simulink model "Example_SOMU_SYNC"  (R2018b)
settings: Solver=FixedStepDiscrete  StartTime=0.0  StopTime=inf  RelTol=1e-3  EnableMultiTasking=on
model workspace: external: MATLAB File (data not in the file)
values from neighbouring files (symbols this model uses):
  kT = acker(Ad,bd,[0.8,0.6])    [aaass.m]
  numOfObj = 5    [aaass.m]    (also in followerGUI.m = max(1,block.DialogPrm(1).Data))
  Td = 0.5    [aaass.m]    (also in controllerSpeed.m = block.DialogPrm(2).Data; followerGUI.m = block.DialogPrm(2).Data; leaderGUI.m = block.DialogPrm(2).Data)
  V = 1./(cT*inv(eye*(2) - Ad+bd*kT)*bd)    [aaass.m]
undefined symbols (not defined in the file or in its folder): Lib_SUMOInterface, MPCController1, sigbuilder_block, SUMU_SIMULINK_SYNC
libraries: simulink x2, Lib_SENSOR x1
settings Model: Creator=michaelstolz  LastModifiedBy=HP
settings SolverCC: AlgebraicLoopSolver=LineSearch
settings DataIOCC: SaveFormat=Array  SaveOutput=off  SignalLogging=off  SaveTime=off
settings OptimizationCC: LifeSpan=inf
settings DebuggingCC: UnderspecifiedInitializationDetection=Classic  MergeDetectMultiDrivingBlocksExec=none  SolverPrmCheckMsg=warning  FcnCallInpInsideContextMsg=warning  SFUnexpectedBacktrackingDiag=warning  SFNoUnconditionalDefaultTransitionDiag=warning  SFExecutionAtInitializationDiag=none
settings HardwareCC: ProdBitPerPointer=32  ProdBitPerSizeT=32  ProdBitPerPtrDiffT=32  ProdLargestAtomicFloat=None  ProdIntDivRoundTo=Undefined  ProdEndianess=Unspecified  ProdWordSize=32  ProdHWDeviceType=32-bit Generic
settings ModelReferenceCC: PropagateSignalLabelsOutOfModel=off
settings SFSimCC: SimUseLocalCustomCode=off
settings RTWCC: RTWUseLocalCustomCode=off
settings CodeAppCC: StateflowObjectComments=on
settings GRTTargetCC: TargetLangStandard=C89/C90 (ANSI)  GeneratePreprocessorConditionals=Disable all
settings ConfigComp: CovMetricSettings=dw  CovHtmlReporting=on  CovSaveCumulativeToWorkspaceVar=on  CovSaveSingleToWorkspaceVar=on  CovExternalEMLEnable=off

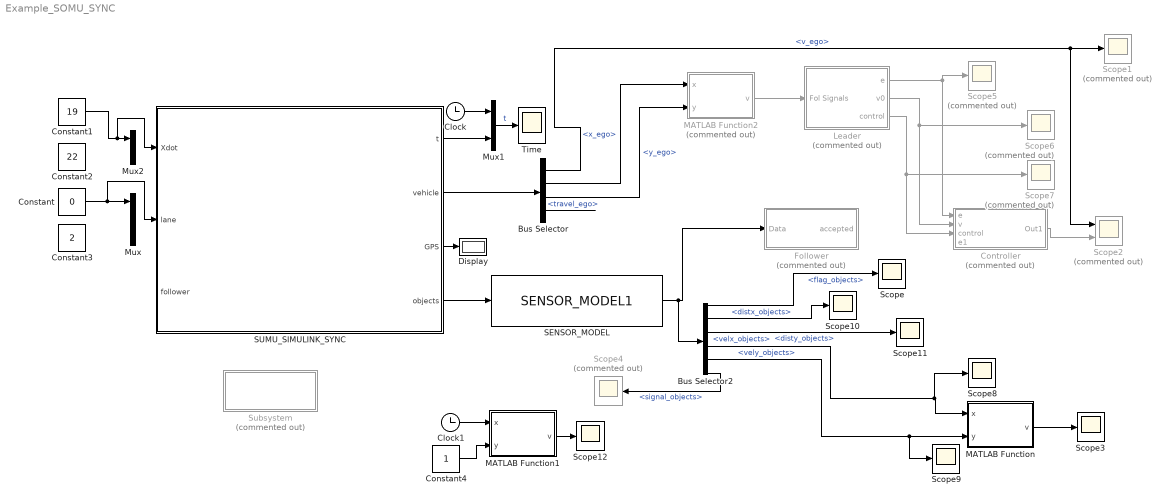
== system Example_SOMU_SYNC ==
  Bus Selector : BusSelector  OutputSignals=v_ego,x_ego,y_ego,travel_ego
  Bus Selector2 : BusSelector  OutputSignals=flag_objects,distx_objects,disty_objects,velx_objects,vely_objects,signal_objects
  Clock : Clock
  Clock1 : Clock
  Constant : Constant  Value=0
  Constant1 : Constant  Value=19
  Constant2 : Constant  Value=22
  Constant3 : Constant  Value=2
  Constant4 : Constant
  Controller : Subsystem  Commented=on
  Display : Display
  Follower : Subsystem  Commented=on
  Leader : Subsystem  Commented=on
  MATLAB Function : MATLAB Function  TreatAsAtomicUnit=on
  MATLAB Function1 : MATLAB Function  TreatAsAtomicUnit=on
  MATLAB Function2 : MATLAB Function  Commented=on  TreatAsAtomicUnit=on
  Mux : Mux  Inputs=3
  Mux1 : Mux  Inputs=2
  Mux2 : Mux  Inputs=3
  SENSOR_MODEL : Lib_SENSOR/SENSOR_MODEL1  NumObjects_=numOfObj  MountX_=[-4,-2,-2]  MountY_=[0,1,-1]  MountA_=[180,90,-90]  SensorModel_=Sector Model  SensorAngle_=[80,100,100]  SensorRange_=[200,20,20]  SensorXY_="{[0   6.5  12.5  20 27.5  35  42.5 47.5 41;  0   7  12  16 19 20  19 10 0 ], [0   6.5  12.5  20 27.5  35  42.5 47.5 41;  0   7  12  16 19 20  19 10 0 ], [0   6.5  12.5  20 27.5  35  42.5 47.5 41;  0   7  12  16 19 20  19 10 0 ]}"  SensorVisibility_=Segmentation  SensorSegmentation_=50  SensorMinVis_=0  SensorType_={'L','L','R'}  NrSensors_=1
  SUMU_SIMULINK_SYNC : Subsystem  AncestorBlock=Lib_SUMOInterface/SUMU_SIMULINK_SYNC  mask(SUMO Simulink Syncronisation){SumoTs_=Td, EgoName_={'ego'}, SumoCfg_=data1\hokkaido.sumocfg, SumoGui_=on, SumoIP_=127.0.0.1, SumoPort_=8873, SumoOptions_=, NumVehicles_=numOfObj, SensorRange_=500, NumTLights_=2}
      mask prompts: SumoTs_ "Sample time for SUMO in [s]"; EgoName_ "Ego vehicle name(s) in SUMO"; SumoCfg_ "SUMO config-file name. (delete for dialog)"; SumoGui_ "Select if the GUI is used or the command line executable."; SumoIP_ "Connection name (default '127.0.0.1')"; SumoPort_ "Port number for SUMO connection (deault 8873)."; SumoOptions_ "Additional command line options for sumo executable."; NumVehicles_ "Maximum number of traffic objects"; SensorRange_ "Detection range [m]. (values <=0 disables range checking)"; NumTLights_ "Maximum number of traffic lights"
      mask help:
      | This Block syncs a vehicle simulation in Simulink with a traffic simulation
      | in SUMO.
      |
      | Syncronisation is performed for one or more vehicle(s) called the
      | "ego"-vehicle(s).
      | The position and velocity information provided from vehicle simulation is
      | send to SUMO to move the corresponding vehicle in the traffic simulation
      | acordingly.
      |
      | Inputs:
      | X     [m] ...... horzintal position of vehicle to sync
      | Y     [m] ...... vertical position of vehicle to sync
      | dX/dt [m/s] .... horizontal velocity of vehicle to sync
      | dY/dt [m/s] .... horizontal velocity of vehicle to sync
      | T     [rad] .... orientation of vehicle to sync
      |                  ( OPTIONAL if sensors are used, otherwise set to NaN )
      | lane  [-] ...... lane of vehicle if in a multilane scenario
      |                  ( currently not used )
      | y_L   [m] ...... lateral offset of vehicle to sync
      |                  ( OPTIONAL if lane assignment shall be done, otherwise 0)
      |
      | Outputs:
      |  * t [s] ....... SUMO simulation time
      |                  (for checking and for traffic light trigger checks)
      |  * vehicle ..... information for ego vehicle(s) within a bus
      |  * GPS   ....... additional GPS information for ego vehicle(s) in a bus
      |  * objects ..... information regarding traffic objects in range in a bus
      |  * signals ..... information regarding traffic lights ahead in a bus
      |
      | Please read the help text for further information.
      mask Help:
      | MASK PARAMETERS:
      | 
      | The following mask parameters can be set, in order to control the behavior of the sync interface:
      | 
      | o) Ego vehicle names as strings in cell array. These names correspond to to the vehicle names in the SUMO config file which should be synced.
      | o) SUMO sample time in [s]: this is the fixed time step SUMO is updated
      | o) SUMO interface IP adress and port number
      | o) SUMO graphical mode activation/diactivation: set wheter to use the gui or command line tool only
      | o) SUMO configuartion file name: better use relative paths for interoperability
      | o) SUMO additional command line parameters: add options to e.g. log something
      | 
      | o) Maximum number of traffic objects to be send at output
      | o) Maximum range around vehicle for traffic objects to be relevant
      | 
      | o) Maximum number of traffic lights to be send at output
      | 
      | POSITION SYNCRONISATION:
      | 
      | Due to several shortcomings of the used TraCi-Interface from SUMO direct position synchronization could not be used in general, therefore
      | indirect synchronization via velocity is used.
      | 
      | Velocity information is used as main syncronization method. Position info is used additionally to correct velocity to improve matching and avoid
      | drifting.
      | Note that setting velocity of the ego-vehicle for synchronization will not in all cases take imidiate effect due to acceleration limits and driver
      | model limitations. However a lot of measures have been taken in order to set the velocity directly:
      |   * min/max acceleration rates have been set to +-1000
      |   * time const of driver model has been set to 0
      |   * speed mode has been set to 0 --> ignoring a lot of speedlimits
      |   * --ignore-accidents has been used in command line
      | 
      | 
      | 
      | INTERFACES:
      | 
      | t : scalar time of SUMO-simulation in seconds.
      | 
      | vehicle : a bus holding ego vehicles informations
      |     * X position [m]
      |     * Y position [m]
      |     * V velocity [m/s]
      |     * T angle [rad] (anticlockwise starting from x)
      |     * D traveled distance [m]
      | 
      | GPS: a bus holding information from FIRST ego car and its road segment
      | 
      | objects: a bus holding information from traffic objects in the given range (mask parameter) of the FIRST ego car. Note the bus signals stay the same, the dimension of each signal will depend on the selected maximum number of traffic objects (mask parameter)
      |  flag_objects : 0=off, 1=on, 2=on and new
      | distx_objects : the distance of the object measured in coordinate system of the FIRST ego vehicle along the x axis
      | disty_objects : the distance of the object measured in coordinate system of the FIRST ego vehicle along the y axis
      | velx_objects : the velocity (absolute!) of the object measured in coordinate system of the FIRST ego vehicle along the x axis
      | vely_objects : the velocity (absolute!) of the object measured in coordinate system of the FIRST ego vehicle along the y axis
      | signal_objects : the signal state of the traffic object. see SUMO documentation for details (brake signal, lane change signal, ...)
      | 
      | signals: a bus holding information from traffic lights ahead of the FIRST ego vehicle. Note the bus signals stay the same, the dimension of each signal will depend on the selected maximum number of traffic lights (mask parameter).
      | flag_signals     : 0=off, 1=on
      | distance_signals : driving distance along the road to the traffic light
      | tswitch_signals  : (absolute) time instance of next switching in seconds
      | phase_signals    : current phase (0 for green, 1 for red)
      | red_signals      : duration of red phase in seconds
      | green_signals    : duration of green phase in seconds
      mask TypeOptions SumoTs_: SIM_SYNC/SumoTs
      mask TypeOptions EgoName_: SIM_SYNC/EgoName
      mask Callback EgoName_:
      | if isempty(get_param(gcb,'EgoName_')),
      |     set_param(gcb, 'EgoName_','{''ego''}');
      | end
      mask TypeOptions SumoCfg_: SIM_SYNC/SumoCfg
      mask Callback SumoCfg_:
      | if isempty(get_param(gcb,'SumoCfg_')),
      |     [myvars.fileName, myvars.filePath] = uigetfile('*.sumocfg','Select a SUMO config File');
      |     if ~isequal(myvars.fileName,0),
      |         set_param(gcb, 'SumoCfg_',fullfile(myvars.filePath,myvars.fileName));
      |     end
      |     clear myvars
      | end
      mask TypeOptions SumoGui_: SIM_SYNC/SumoGui
      mask TypeOptions SumoIP_: SIM_SYNC/SumoIP
      mask Callback SumoIP_:
      | if isempty(get_param(gcb,'SumoIP_')),
      |     set_param(gcb, 'SumoIP_','127.0.0.1');
      | end
      mask TypeOptions SumoPort_: SIM_SYNC/SumoPort
      mask Callback SumoPort_:
      | if isempty(get_param(gcb,'SumoPort_')),
      |     set_param(gcb, 'SumoPort_','8873');
      | end
      mask TypeOptions SumoOptions_: SIM_SYNC/SumoOptions
      mask TypeOptions NumVehicles_: SIM_SYNC/NumVehicles
      mask Callback NumVehicles_:
      | if isempty(get_param(gcb,'NumVehicles_')),
      |     set_param(gcb, 'NumVehicles_','0');
      | end
      mask TypeOptions SensorRange_: SIM_SYNC/SensorRange
      mask TypeOptions NumTLights_: SIM_SYNC/NumTLights
      mask Callback NumTLights_:
      | if isempty(get_param(gcb,'NumTLights_')),
      |     set_param(gcb, 'NumTLights_','0');
      | end
      mask DialogControl ParameterTabVar0 Prompt: SIMULATION
      mask DialogControl ParameterTabVar01 Prompt: SUMO
      mask DialogControl ParameterTabVar012 Prompt: OBJECTS
      mask DialogControl ParameterTabVar0123 Prompt: SIGNALS
      mask Display:
      | text(.5,.8,'\fontname{palatino}\fontsize{15}\bf Simulink-SUMO SYNC',...
      |       'HorizontalAlignment','center','texmode','on');
      | text(.5,.6,['sample rate = ',sprintf('%4.2f [s]',SumoTs_)],...
      |       'HorizontalAlignment','center','texmode','on');
      | text(.5,.4,['ego vehicle name : ',sprintf('"%s" ',EgoName_{:})],...
      |       'HorizontalAlignment','center','texmode','off');
      | text(.5,.2,sprintf('"%s"',SumoCfg_),...
      |       'HorizontalAlignment','center','texmode','off');
      | port_label('input',1,'vel [m/s]');
      | 
      | port_label('input',2,'lane  [-]');
      | 
      | port_label('input',3,'follower  [-]');
      | 
      | 
      | port_label('output',1,'t');
      | port_label('output',2,'vehicle');
      | port_label('output',3,'GPS');
      | port_label('output',4,sprintf('%d objects',NumVehicles_));
  Scope{,3,8..12} (7 alike) : Scope
  Scope{1,4..7} (5 alike) : Scope  Commented=on
  Scope2 : Scope  Commented=on  NumInputPorts=2
  Subsystem : Subsystem  Commented=on
  Time : Scope
  wires:
  Mux1/1 -> Time/1  "t"
  Clock/1 -> Mux1/1
  SUMU_SIMULINK_SYNC/1(t) -> Mux1/2
  Bus Selector/3 -> MATLAB Function2/2(y)  "<y_ego>"
  Bus Selector/1 -> Scope2/1, Scope1/1  "<v_ego>"
  Bus Selector/4 -> ?  "<travel_ego>"
  SUMU_SIMULINK_SYNC/3(GPS) -> Display/1
  Bus Selector2/2 -> Scope10/1  "<distx_objects>"
  Bus Selector2/1 -> Scope/1  "<flag_objects>"
  Bus Selector2/3 -> Scope11/1  "<disty_objects>"
  Bus Selector2/6 -> Scope4/1  "<signal_objects>"
  Bus Selector2/5 -> Scope9/1, MATLAB Function/2(y)  "<vely_objects>"
  Bus Selector2/4 -> Scope8/1, MATLAB Function/1(x)  "<velx_objects>"
  SENSOR_MODEL/1 -> Bus Selector2/1, Follower/1(Data)
  SUMU_SIMULINK_SYNC/4(objects) -> SENSOR_MODEL/1
  Bus Selector/2 -> MATLAB Function2/1(x)  "<x_ego>"
  SUMU_SIMULINK_SYNC/2(vehicle) -> Bus Selector/1
  Controller/1(Out1) -> Scope2/2
  MATLAB Function/1(v) -> Scope3/1
  Leader/1(e) -> Scope5/1, Controller/1(e)
  Leader/2(v0) -> Scope6/1, Controller/2(v)
  Leader/3(control) -> Scope7/1, Controller/3(control)
  Constant1/1 -> SUMU_SIMULINK_SYNC/1(Xdot), Mux2/1
  MATLAB Function2/1(v) -> Leader/1(Fol Signals)
  Constant/1 -> SUMU_SIMULINK_SYNC/2(lane), Mux/1
  Clock1/1 -> MATLAB Function1/1(x)
  MATLAB Function1/1(v) -> Scope12/1
  Constant4/1 -> MATLAB Function1/2(y)

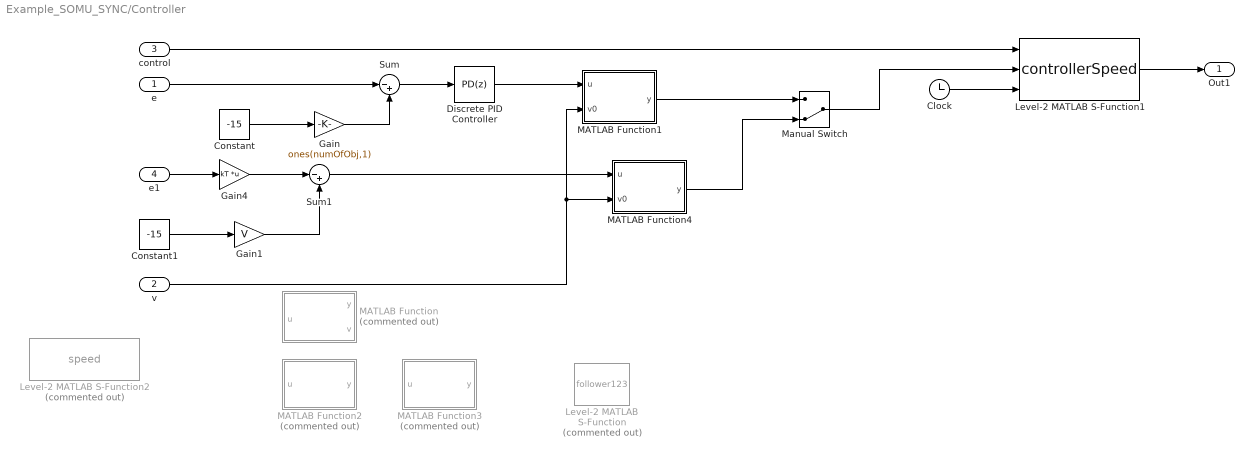
== system Example_SOMU_SYNC/Controller ==
  e : Inport
  v : Inport  Port=2
  control : Inport  Port=3
  e1 : Inport  Port=4
  Clock : Clock
  Constant : Constant  Value=-15
  Constant1 : Constant  Value=-15
  Discrete PID Controller : simulink/Continuous/PID Controller  Controller=PD  Form=Parallel  TimeDomain=Discrete-time  SampleTime=Td  IntegratorMethod=Forward Euler  FilterMethod=Forward Euler  ControllerParametersSource=internal  P=0.4  I=1  D=1  UseFilter=off  N=50  TunerSelectOption=Transfer Function Based (PID Tuner App)  InitialConditionSource=internal  InitialConditionForIntegrator=0  InitialConditionForFilter=0  DifferentiatorICPrevScaledInput=0  ExternalReset=none  TrackingMode=off  Kt=1  LimitOutput=on  UpperSaturationLimit=10  LowerSaturationLimit=-10  LinearizeAsGain=off  AntiWindupMode=none  Kb=1  POutMin=[]  POutMax=[]  IOutMin=[]  IOutMax=[]  DOutMin=[]  DOutMax=[]  NOutMin=[]  NOutMax=[]  SumOutMin=[]  SumOutMax=[]  SaturationOutMin=[]  SaturationOutMax=[]  PParamMin=[]  PParamMax=[]  IParamMin=[]  IParamMax=[]  DParamMin=[]  DParamMax=[]  NParamMin=[]  NParamMax=[]  KbParamMin=[]  KbParamMax=[]  KtParamMin=[]  KtParamMax=[]  KbOutMin=[]  KbOutMax=[]  KtOutMin=[]  KtOutMax=[]  IntegratorOutMin=[]  IntegratorOutMax=[]  FilterOutMin=[]  FilterOutMax=[]  SumI1OutMin=[]  SumI1OutMax=[]  SumI2OutMin=[]  SumI2OutMax=[]  SumI3OutMin=[]  SumI3OutMax=[]  SumI4OutMin=[]  SumI4OutMax=[]  SumDOutMin=[]  SumDOutMax=[]  DifferentiatorOutMin=[]  DifferentiatorOutMax=[]  FilterDiffOutCoefMin=[]  FilterDiffOutCoefMax=[]  ReciprocalOutMin=[]  ReciprocalOutMax=[]  SumDenOutMin=[]  SumDenOutMax=[]  SumNumOutMin=[]  SumNumOutMax=[]  DivideOutMin=[]  DivideOutMax=[]  IntegratorContinuousStateAttributes=''  IntegratorStateMustResolveToSignalObject=off  IntegratorRTWStateStorageClass=Auto  FilterContinuousStateAttributes=''  FilterStateMustResolveToSignalObject=off  FilterRTWStateStorageClass=Auto  ParallelPVariant=InternalParameters  IdealPVariant=Disabled  IVariant=Disabled  DVariant=InternalParameters  IntegratorVariant=Disabled  SatVariant=Enabled  AWVariant=Disabled  PCopyVariant=Disabled  TRVariant=Disabled  FdbkBlocksVariant=Forward  IdealPFdbkVariant=Disabled  SatFdbkVariant=Disabled  DerivativeFilterVariant=Differentiator  NVariant=Passthrough  NCopyVariant=Disabled_SignalSpec  FilterICVariant=InternalICsDifferentiator  IntegratorICVariant=Disabled  ExternalResetVariant=Disabled  TRSumVariant=Passthrough  SumFdbkVariant=Disabled  SumVariant=Sum_PD
  Gain : Gain  Gain=ones(numOfObj,1)
  Gain1 : Gain  Gain=V
  Gain4 : Gain  Gain=kT  Multiplication=Matrix(K*u)
  Level-2 MATLAB S-Function : M-S-Function  Commented=on  FunctionName=follower123  Parameters=numOfObj
  Level-2 MATLAB S-Function1 : M-S-Function  FunctionName=controllerSpeed  Parameters=numOfObj,Td
  Level-2 MATLAB S-Function2 : M-S-Function  Commented=on  FunctionName=speed  Parameters=numOfObj
  MATLAB Function : MATLAB Function  Commented=on  TreatAsAtomicUnit=on
  MATLAB Function1 : MATLAB Function  TreatAsAtomicUnit=on
  MATLAB Function2 : MATLAB Function  Commented=on  TreatAsAtomicUnit=on
  MATLAB Function3 : MATLAB Function  Commented=on  TreatAsAtomicUnit=on
  MATLAB Function4 : MATLAB Function  TreatAsAtomicUnit=on
  Manual Switch : ManualSwitch  CurrentSetting=0
  Sum : Sum  Inputs=|-+
  Sum1 : Sum  Inputs=|-+
  Out1 : Outport
  wires:
  e/1 -> Sum/1
  Constant/1 -> Gain/1
  Sum/1 -> Discrete PID Controller/1
  Discrete PID Controller/1 -> MATLAB Function1/1(u)
  v/1 -> MATLAB Function4/2(v0), MATLAB Function1/2(v0)
  MATLAB Function1/1(y) -> Manual Switch/1
  Level-2 MATLAB S-Function1/1 -> Out1/1
  control/1 -> Level-2 MATLAB S-Function1/1
  Gain/1 -> Sum/2
  Clock/1 -> Level-2 MATLAB S-Function1/3
  Manual Switch/1 -> Level-2 MATLAB S-Function1/2
  MATLAB Function4/1(y) -> Manual Switch/2
  e1/1 -> Gain4/1
  Gain4/1 -> Sum1/1
  Constant1/1 -> Gain1/1
  Gain1/1 -> Sum1/2
  Sum1/1 -> MATLAB Function4/1(u)

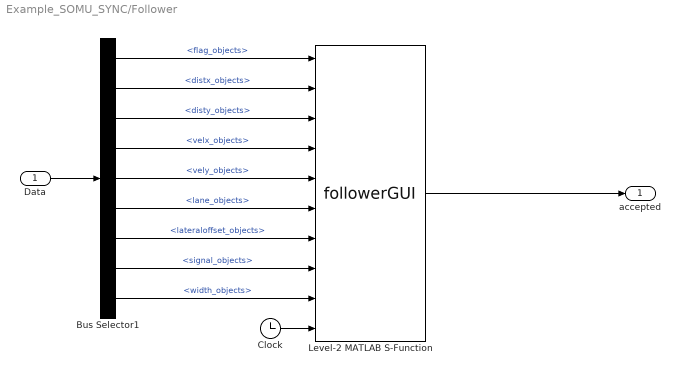
== system Example_SOMU_SYNC/Follower ==
  Data : Inport
  Bus Selector1 : BusSelector  OutputSignals=flag_objects,distx_objects,disty_objects,velx_objects,vely_objects,lane_objects,lateraloffset_objects,signal_objects,width_objects
  Clock : Clock
  Level-2 MATLAB S-Function : M-S-Function  FunctionName=followerGUI  Parameters=numOfObj,Td
  accepted : Outport
  wires:
  Level-2 MATLAB S-Function/1 -> accepted/1
  Data/1 -> Bus Selector1/1
  Bus Selector1/9 -> Level-2 MATLAB S-Function/9  "<width_objects>"
  Bus Selector1/8 -> Level-2 MATLAB S-Function/8  "<signal_objects>"
  Bus Selector1/7 -> Level-2 MATLAB S-Function/7  "<lateraloffset_objects>"
  Bus Selector1/6 -> Level-2 MATLAB S-Function/6  "<lane_objects>"
  Bus Selector1/5 -> Level-2 MATLAB S-Function/5  "<vely_objects>"
  Bus Selector1/4 -> Level-2 MATLAB S-Function/4  "<velx_objects>"
  Bus Selector1/3 -> Level-2 MATLAB S-Function/3  "<disty_objects>"
  Bus Selector1/2 -> Level-2 MATLAB S-Function/2  "<distx_objects>"
  Clock/1 -> Level-2 MATLAB S-Function/10
  Bus Selector1/1 -> Level-2 MATLAB S-Function/1  "<flag_objects>"

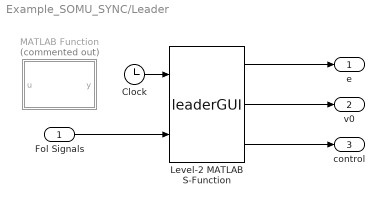
== system Example_SOMU_SYNC/Leader ==
  Fol Signals : Inport
  Clock : Clock
  Level-2 MATLAB S-Function : M-S-Function  FunctionName=leaderGUI  Parameters=numOfObj,Td
  MATLAB Function : MATLAB Function  Commented=on  TreatAsAtomicUnit=on
  e : Outport
  v0 : Outport  Port=2
  control : Outport  Port=3
  wires:
  Fol Signals/1 -> Level-2 MATLAB S-Function/2
  Level-2 MATLAB S-Function/1 -> e/1
  Clock/1 -> Level-2 MATLAB S-Function/1
  Level-2 MATLAB S-Function/2 -> v0/1
  Level-2 MATLAB S-Function/3 -> control/1

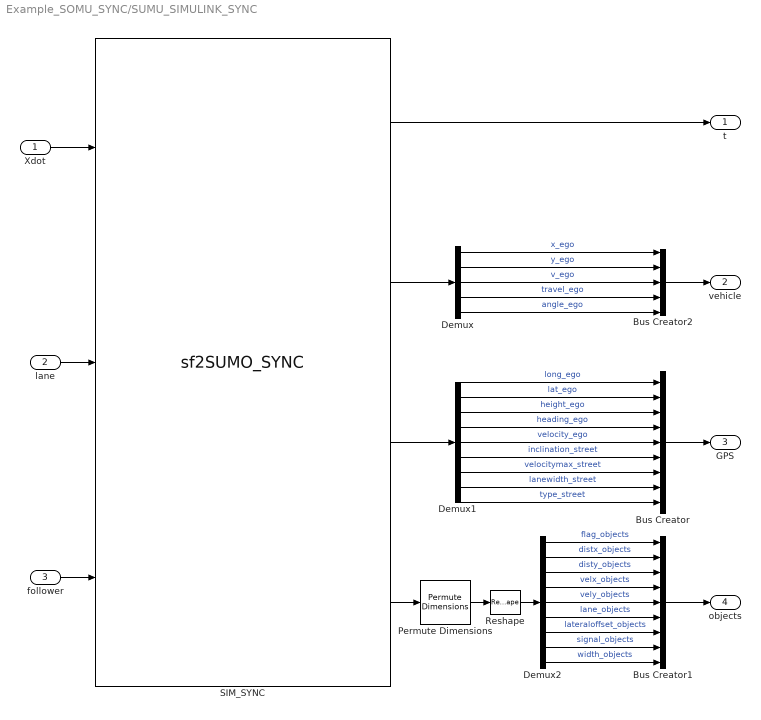
== system Example_SOMU_SYNC/SUMU_SIMULINK_SYNC ==
  Xdot : Inport
  lane : Inport  Port=2
  follower : Inport  Port=3
  Bus Creator : BusCreator  Inputs=9
  Bus Creator1 : BusCreator  Inputs=9
  Bus Creator2 : BusCreator  Inputs=5
  Demux : Demux  Outputs=5
  Demux1 : Demux  Outputs=9
  Demux2 : Demux  Outputs=[-1,-1,-1,-1,-1,-1,-1,-1,-1]
  Permute Dimensions : PermuteDimensions
  Reshape : Reshape
  SIM_SYNC : M-S-Function  FunctionName=sf2SUMO_SYNC  Parameters=SumoTs,EgoName,NumVehicles,SumoCfg,SumoIP,SumoPort,SumoGui,SumoOptions,NumTLights,SensorRange  mask(SUMO Simulink Syncronisation){SumoTs=SumoTs_, EgoName=EgoName_, SumoPort=SumoPort_, SumoIP=127.0.0.1, SumoCfg=data1\hokkaido.sumocfg, SumoGui=on, SumoOptions=, NumVehicles=NumVehicles_, SensorRange=SensorRange_, NumTLights=NumTLights_}
      mask prompts: SumoTs "Sample time for SUMO in [s]"; EgoName "Ego vehicle name(s) in SUMO ( default {'ego'} )"; SumoPort "Port number for SUMO connection (default 8873)"; SumoIP "Connection name (default: '127.0.0.1')"; SumoCfg "Full SUMO config-file name"; SumoGui "Select if the GUI is used or the command line tool."; SumoOptions "Additional command line options for SUMO:"; NumVehicles "Maximum number of traffic objects."; SensorRange "Detection range [m]"; NumTLights "Maximum number of traffic lights"
      mask Callback EgoName:
      | if isempty(get_param(gcb,'EgoName')),
      |     set_param(gcb, 'EgoName','{''ego''}');
      | end
      mask Callback SumoPort:
      | if isempty(get_param(gcb,'SumoPort')),
      |     set_param(gcb, 'SumoPort','8873');
      | end
      mask Callback SumoIP:
      | if isempty(get_param(gcb,'SumoIP')),
      |     set_param(gcb, 'SumoIP','127.0.0.1');
      | end
      mask Callback SumoCfg:
      | if isempty(get_param(gcb,'SumoCfg')),
      |     [myvars.fileName, myvars.filePath] = uigetfile('*.sumocfg','Select a SUMO config File');
      |     if ~isequal(myvars.fileName,0),
      |         set_param(gcb, 'SumoCfg',fullfile(myvars.filePath,myvars.fileName));
      |     end
      |     clear myvars
      | end
      mask DialogControl ParameterTabVar0 Prompt: SIMULATION
      mask DialogControl ParameterTabVar01 Prompt: SUMO
      mask DialogControl ParameterTabVar012 Prompt: SENSORS
      mask DialogControl ParameterTabVar0123 Prompt: TRAFFIC LIGHTS
      mask Display:
      | text(.5,.8,'\fontname{palatino}\fontsize{15}\bf Simulink-SUMO SYNC',...
      |       'HorizontalAlignment','center','texmode','on');
      | text(.5,.6,['sample rate = ',sprintf('%4.2f [s]',SumoTs)],...
      |       'HorizontalAlignment','center','texmode','on');
      | text(.5,.4,['ego vehicle name : ',sprintf('"%s" ',EgoName{:})],...
      |       'HorizontalAlignment','center','texmode','off');
      | text(.5,.2,sprintf('"%s"',SumoCfg),...
      |       'HorizontalAlignment','center','texmode','off');
      | 
      | port_label('input',1,'ds/dt [m/s]');
      | 
      | port_label('input',2,'lane  [-]');
      | 
      | 
      | port_label('output',1,'t');
      | port_label('output',2,'vehicle');
      | port_label('output',3,'GPS');
      | port_label('output',4,sprintf('%d objects',NumVehicles));
  t : Outport
  vehicle : Outport  Port=2
  GPS : Outport  Port=3
  objects : Outport  Port=4
  wires:
  Demux2/9 -> Bus Creator1/9  "width_objects"
  SIM_SYNC/2 -> Demux/1
  Demux/2 -> Bus Creator2/2  "y_ego"
  Demux/1 -> Bus Creator2/1  "x_ego"
  Demux/3 -> Bus Creator2/3  "v_ego"
  SIM_SYNC/3 -> Demux1/1
  SIM_SYNC/4 -> Permute Dimensions/1
  Demux1/1 -> Bus Creator/1  "long_ego"
  Demux1/2 -> Bus Creator/2  "lat_ego"
  Demux1/3 -> Bus Creator/3  "height_ego"
  Demux1/4 -> Bus Creator/4  "heading_ego"
  Demux1/5 -> Bus Creator/5  "velocity_ego"
  Demux1/6 -> Bus Creator/6  "inclination_street"
  Demux1/7 -> Bus Creator/7  "velocitymax_street"
  Demux1/8 -> Bus Creator/8  "lanewidth_street"
  Demux1/9 -> Bus Creator/9  "type_street"
  Demux2/1 -> Bus Creator1/1  "flag_objects"
  Demux2/2 -> Bus Creator1/2  "distx_objects"
  Demux2/3 -> Bus Creator1/3  "disty_objects"
  Demux2/4 -> Bus Creator1/4  "velx_objects"
  Demux2/5 -> Bus Creator1/5  "vely_objects"
  Demux2/6 -> Bus Creator1/6  "lane_objects"
  Demux2/7 -> Bus Creator1/7  "lateraloffset_objects"
  Demux2/8 -> Bus Creator1/8  "signal_objects"
  Reshape/1 -> Demux2/1
  Permute Dimensions/1 -> Reshape/1
  Demux/4 -> Bus Creator2/4  "travel_ego"
  Demux/5 -> Bus Creator2/5  "angle_ego"
  SIM_SYNC/1 -> t/1
  Xdot/1 -> SIM_SYNC/1
  Bus Creator2/1 -> vehicle/1
  Bus Creator/1 -> GPS/1
  lane/1 -> SIM_SYNC/2
  Bus Creator1/1 -> objects/1
  follower/1 -> SIM_SYNC/3

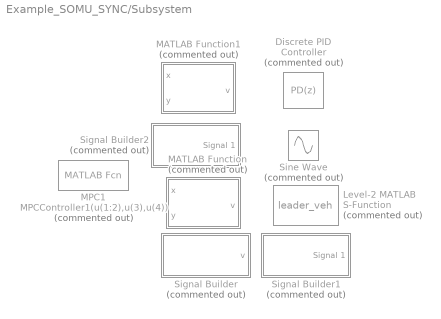
== system Example_SOMU_SYNC/Subsystem ==
  Discrete PID Controller : simulink/Continuous/PID Controller  Commented=on  Controller=PD  Form=Parallel  TimeDomain=Discrete-time  SampleTime=0.5  IntegratorMethod=Forward Euler  FilterMethod=Forward Euler  ControllerParametersSource=internal  P=0.2389  I=1  D=0.05971  UseFilter=off  N=50  TunerSelectOption=Transfer Function Based (PID Tuner App)  InitialConditionSource=internal  InitialConditionForIntegrator=0  InitialConditionForFilter=0  DifferentiatorICPrevScaledInput=0  ExternalReset=none  TrackingMode=off  Kt=1  LimitOutput=off  UpperSaturationLimit=inf  LowerSaturationLimit=-inf  LinearizeAsGain=off  AntiWindupMode=none  Kb=1  POutMin=[]  POutMax=[]  IOutMin=[]  IOutMax=[]  DOutMin=[]  DOutMax=[]  NOutMin=[]  NOutMax=[]  SumOutMin=[]  SumOutMax=[]  SaturationOutMin=[]  SaturationOutMax=[]  PParamMin=[]  PParamMax=[]  IParamMin=[]  IParamMax=[]  DParamMin=[]  DParamMax=[]  NParamMin=[]  NParamMax=[]  KbParamMin=[]  KbParamMax=[]  KtParamMin=[]  KtParamMax=[]  KbOutMin=[]  KbOutMax=[]  KtOutMin=[]  KtOutMax=[]  IntegratorOutMin=[]  IntegratorOutMax=[]  FilterOutMin=[]  FilterOutMax=[]  SumI1OutMin=[]  SumI1OutMax=[]  SumI2OutMin=[]  SumI2OutMax=[]  SumI3OutMin=[]  SumI3OutMax=[]  SumI4OutMin=[]  SumI4OutMax=[]  SumDOutMin=[]  SumDOutMax=[]  DifferentiatorOutMin=[]  DifferentiatorOutMax=[]  FilterDiffOutCoefMin=[]  FilterDiffOutCoefMax=[]  ReciprocalOutMin=[]  ReciprocalOutMax=[]  SumDenOutMin=[]  SumDenOutMax=[]  SumNumOutMin=[]  SumNumOutMax=[]  DivideOutMin=[]  DivideOutMax=[]  IntegratorContinuousStateAttributes=''  IntegratorStateMustResolveToSignalObject=off  IntegratorRTWStateStorageClass=Auto  FilterContinuousStateAttributes=''  FilterStateMustResolveToSignalObject=off  FilterRTWStateStorageClass=Auto  ParallelPVariant=InternalParameters  IdealPVariant=Disabled  IVariant=Disabled  DVariant=InternalParameters  IntegratorVariant=Disabled  SatVariant=Disabled  AWVariant=Disabled  PCopyVariant=Disabled  TRVariant=Disabled  FdbkBlocksVariant=Forward  IdealPFdbkVariant=Disabled  SatFdbkVariant=Disabled  DerivativeFilterVariant=Differentiator  NVariant=Passthrough  NCopyVariant=Disabled_SignalSpec  FilterICVariant=InternalICsDifferentiator  IntegratorICVariant=Disabled  ExternalResetVariant=Disabled  TRSumVariant=Passthrough  SumFdbkVariant=Disabled  SumVariant=Sum_PD
  Level-2 MATLAB S-Function : M-S-Function  Commented=on  FunctionName=leader_veh
  MATLAB Function : MATLAB Function  Commented=on  TreatAsAtomicUnit=on
  MATLAB Function1 : MATLAB Function  Commented=on  TreatAsAtomicUnit=on
  MPC1 : MATLABFcn  Commented=on  MATLABFcn=MPCController1(u(1:2),u(3),u(4))
  Signal Builder : Subsystem  Tag=STV Subsys  Commented=on  LoadFcn=sigbuilder_block('load');  StartFcn=sigbuilder_block('start');  StopFcn=sigbuilder_block('stop');  ClipboardFcn=sigbuilder_block('clipboard');  mask(Sigbuilder block){tuvar=[0:10]}
      mask help: Simulink:masks:SigbuilderBlock_MD
      mask init:
      | if ~strcmp(get_param(bdroot(gcbh),'SimulationStatus'),'stopped') tuvar = sigbuilder_block('maskInit'); end
      settings: CopyFcn=sigbuilder_block('copy');  DeleteFcn=sigbuilder_block('delete');  ModelCloseFcn=sigbuilder_block('modelClose');  PreSaveFcn=sigbuilder_block('preSave');  PauseFcn=sigbuilder_block('pause');  ContinueFcn=sigbuilder_block('continue');  NameChangeFcn=sigbuilder_block('namechange');  OpenFcn=sigbuilder_block('open',[435.75 150.75 549 361.5 ]);  CloseFcn=sigbuilder_block('close');
      mask Display: plot(0, 0, 100, 100,[2, 2, 32, 32, 2], [68, 8, 8, 68, 68],[32, 2], [38, 38], [32, 19, 2],[53, 60, 44], [32, 17, 17, 2],[16, 16, 31, 31]);txt = getActiveGroup(gcbh);text(2, 100, txt,'verticalAlignment', 'top');
  Signal Builder1 : Subsystem  Tag=STV Subsys  Commented=on  LoadFcn=sigbuilder_block('load');  StartFcn=sigbuilder_block('start');  StopFcn=sigbuilder_block('stop');  ClipboardFcn=sigbuilder_block('clipboard');  mask(Sigbuilder block){tuvar=[0:10]}
      mask help: Simulink:masks:SigbuilderBlock_MD
      mask init:
      | if ~strcmp(get_param(bdroot(gcbh),'SimulationStatus'),'stopped') tuvar = sigbuilder_block('maskInit'); end
      settings: CopyFcn=sigbuilder_block('copy');  DeleteFcn=sigbuilder_block('delete');  ModelCloseFcn=sigbuilder_block('modelClose');  PreSaveFcn=sigbuilder_block('preSave');  PauseFcn=sigbuilder_block('pause');  ContinueFcn=sigbuilder_block('continue');  NameChangeFcn=sigbuilder_block('namechange');  OpenFcn=sigbuilder_block('open',[437.25 199.5 550.5 399.75 ]);  CloseFcn=sigbuilder_block('close');
      mask Display: plot(0, 0, 100, 100,[2, 2, 32, 32, 2], [68, 8, 8, 68, 68],[32, 2], [38, 38], [32, 19, 2],[53, 60, 44], [32, 17, 17, 2],[16, 16, 31, 31]);txt = getActiveGroup(gcbh);text(2, 100, txt,'verticalAlignment', 'top');
  Signal Builder2 : Subsystem  Tag=STV Subsys  Commented=on  LoadFcn=sigbuilder_block('load');  StartFcn=sigbuilder_block('start');  StopFcn=sigbuilder_block('stop');  ClipboardFcn=sigbuilder_block('clipboard');  mask(Sigbuilder block){tuvar=[0:10]}
      mask help: Simulink:masks:SigbuilderBlock_MD
      mask init:
      | if ~strcmp(get_param(bdroot(gcbh),'SimulationStatus'),'stopped') tuvar = sigbuilder_block('maskInit'); end
      settings: CopyFcn=sigbuilder_block('copy');  DeleteFcn=sigbuilder_block('delete');  ModelCloseFcn=sigbuilder_block('modelClose');  PreSaveFcn=sigbuilder_block('preSave');  PauseFcn=sigbuilder_block('pause');  ContinueFcn=sigbuilder_block('continue');  NameChangeFcn=sigbuilder_block('namechange');  OpenFcn=sigbuilder_block('open',[6 30 1012.5 447.75 ]);  CloseFcn=sigbuilder_block('close');
      mask Display: plot(0, 0, 100, 100,[2, 2, 32, 32, 2], [68, 8, 8, 68, 68],[32, 2], [38, 38], [32, 19, 2],[53, 60, 44], [32, 17, 17, 2],[16, 16, 31, 31]);txt = getActiveGroup(gcbh);text(2, 100, txt,'verticalAlignment', 'top');
  Sine Wave : Sin  Commented=on  Bias=20  Frequency=0.1  SampleTime=0

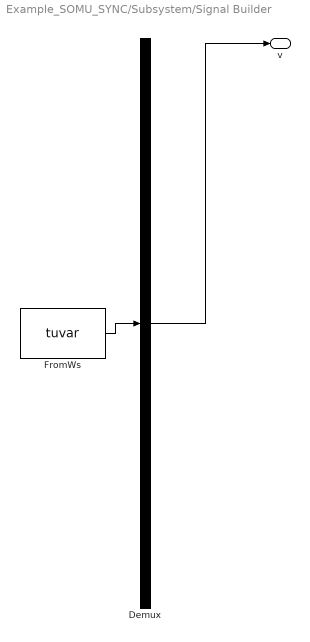
== system Example_SOMU_SYNC/Subsystem/Signal Builder ==
  Demux : Demux  Tag=STV Demux  Outputs=1
  FromWs : FromWorkspace  Tag=STV FromWs  VariableName=tuvar  SampleTime=0
      SigBuilderData=|
      | common.afterFinalStr = 'Extrapolate'
      | common.sampleTime = 0
      | dataSet.timeRange = [0 10]
      | dataSet.name = 'Group 1'
      | sbobj.Groups.Name = 'Group 1'
      | sbobj.Groups.Signals.Name = 'v'
      | sbobj.Groups.Signals.XData = [0 4.8 5 6 6.5 6.5 10]
      | sbobj.Groups.Signals.YData = [20 20 0 0 15 14.9 14.9]
  v : Outport  Tag=STV Outport
  wires:
  Demux/1 -> v/1
  FromWs/1 -> Demux/1

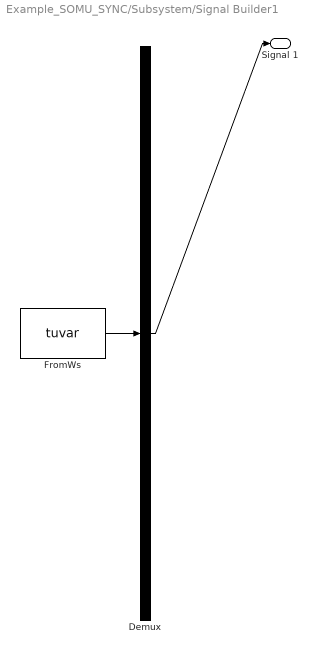
== system Example_SOMU_SYNC/Subsystem/Signal Builder1 ==
  Demux : Demux  Tag=STV Demux  Outputs=1
  FromWs : FromWorkspace  Tag=STV FromWs  VariableName=tuvar  SampleTime=0
      SigBuilderData=|
      | common.afterFinalStr = 'Extrapolate'
      | common.sampleTime = 0
      | dataSet.timeRange = [0 100]
      | dataSet.name = 'Group 1'
      | sbobj.Groups.Name = 'Group 1'
      | sbobj.Groups.Signals.Name = 'Signal 1'
      | sbobj.Groups.Signals.XData = [0 78.6 78.6 91.4 91.4 93 93 94.2 94.2 100]
      | sbobj.Groups.Signals.YData = [0 0 1 1 0 0 1 1 0 0]
      | sbobj.Groups.TimeRange = [0 100]
  Signal 1 : Outport  Tag=STV Outport
  wires:
  FromWs/1 -> Demux/1
  Demux/1 -> Signal 1/1

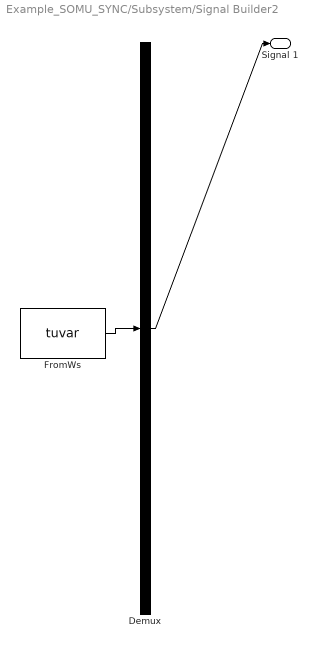
== system Example_SOMU_SYNC/Subsystem/Signal Builder2 ==
  Demux : Demux  Tag=STV Demux  Outputs=1
  FromWs : FromWorkspace  Tag=STV FromWs  VariableName=tuvar  SampleTime=0
      SigBuilderData=|
      | common.afterFinalStr = 'Extrapolate'
      | common.sampleTime = 0
      | dataSet.timeRange = [0 500]
      | dataSet.name = 'Group 1'
      | sbobj.Groups.Name = 'Group 1'
      | sbobj.Groups.Signals.Name = 'Signal 1'
      | sbobj.Groups.Signals.XData = [0 200 200 300 400 500]
      | sbobj.Groups.Signals.YData = [20 20 20 4 8 8]
      | sbobj.Groups.TimeRange = [0 500]
  Signal 1 : Outport  Tag=STV Outport
  wires:
  FromWs/1 -> Demux/1
  Demux/1 -> Signal 1/1

== matlab function Example_SOMU_SYNC/Subsystem/MATLAB Function1 ==
  data: x input; v output; y input
function v = fcn(x,y)

v = -sqrt(x.^2 + y.^2) + 4;

== matlab function Example_SOMU_SYNC/Subsystem/MATLAB Function ==
  data: x input; v output; y input
function v = fcn(x,y)

v = sqrt(x.^2 + y.^2);

== matlab function Example_SOMU_SYNC/MATLAB Function2 ==
  data: x input; v output; y input
function v = fcn(x,y)

v = sqrt(x.^2 + y.^2);

== matlab function Example_SOMU_SYNC/Leader/MATLAB Function ==
  data: u input; y output
function y = fcn(u)

if traci.vehicle.getSignals('x') == 13
    traci.vehicle.setSignals('ego',12);
end
y = u;

== matlab function Example_SOMU_SYNC/Controller/MATLAB Function ==
  data: u input; y output; v output
function [y ,v] = fcn(u)

global IDsVeh;

if u(find(strcmp({'x'}, IDsVeh))) == 1
    s_leader   = traci.vehicle.getDistance('ego');
    s_follower = traci.vehicle.getDistance('x');
    y = s_follower - s_leader;
    v = traci.vehicle.getSpeed{'x'};
end

== matlab function Example_SOMU_SYNC/Controller/MATLAB Function1 ==
  data: u input; y output; v0 input; Td parameter
function y = fcn(u,v0,Td)

y = u*Td+v0;

== matlab function Example_SOMU_SYNC/Controller/MATLAB Function2 ==
  data: u input; y output
function y = fcn(u)
traci.vehicle.setSpeed('x',u);
y = u;

== matlab function Example_SOMU_SYNC/MATLAB Function ==
  data: x input; v output; y input
function v = fcn(x,y)

v = sqrt(x.^2 + y.^2);

== matlab function Example_SOMU_SYNC/Controller/MATLAB Function3 ==
  data: u input; y output
function y = fcn(u)
global IDsVeh;
y = u(find(strcmp({'x'}, IDsVeh)));

== matlab function Example_SOMU_SYNC/MATLAB Function1 ==
  data: x input; v output; y input
function v = fcn(x,y)
v = 0;
if x > 5
    v = traci.vehicle.getSpeed('ego');
end

== matlab function Example_SOMU_SYNC/Controller/MATLAB Function4 ==
  data: u input; y output; v0 input; Td parameter
function y = fcn(u,v0,Td)

y = u*Td+v0;
